simulink model "IDC_OS"  (R2023b)
settings: Solver=FixedStepAuto  StartTime=0.0  StopTime=9  FixedStep=sampleTime  RelTol=1e-3
values from neighbouring files (symbols this model uses):
  initialguess = robot.homeConfiguration    [IDC_OS.m]
  K_D = 0*eye(n_joints)    [IDC_OS.m]
  K_P = 0*eye(n_joints)    [IDC_OS.m]
  n_joints = 6    [IDC_OS.m]
  robot = loadrobot("universalUR5")    [IDC_OS.m]
  t0 = 0    [IDC_OS.m]
  t1 = 5    [IDC_OS.m]
  t2 = 10    [IDC_OS.m]
  t3 = 100    [IDC_OS.m]
  weights = transpose([0.1, 0.1, 0.1, 1, 1, 1])    [IDC_OS.m]
  x0_pose = trvec2tform([x0(1), x0(2), x0(3)]) * eul2tform([x0(4), x0(5), x0(6)])    [IDC_OS.m]
  xd = zeros(n_joints,1)    [IDC_OS.m]
undefined symbols (not defined in the file or in its folder): x1_pose, x2_pose
libraries: robotmaniplib x8
(part 2 of 2)

== matlab function IDC_OS/J_A^(-1)(q)*[...]/Analytical Jacobian/Analytical from Geometric ==
  data: geomJ input; Ja output; angles input
function Ja = JacobAnFromGeomWrapper(geomJ,angles)
% For T^-1 matrix using RPY i.e., z(r) y(p) x(y) wrt to the current frame

T = rpy2Tmatrix(angles);

Tinv = inv(T);

% Following matlab convention (Jo is on top of Jp)
Ja = [Tinv,zeros(3);zeros(3),eye(3)] * geomJ;

% In standard convention one would have:
% analytJ = [eye(3),zeros(3);zeros(3),Tinv] * geomJ;

== matlab function IDC_OS/J_A^(-1)(q)*[...]/Analytical Jacobian/Direct Kinematics/get RPY angles ==
  data: R input; rpy output
function rpy = rpyWrap(R)
%rpy = getRPYanglesFromR(R);
[rpy, ~] = eulerInverseProblem(R,'zyx','current');

== matlab function IDC_OS/J_A(q)*q./Analytical Jacobian/Direct Kinematics/get RPY angles ==
  data: R input; rpy output
function rpy = rpyWrap(R)
%rpy = getRPYanglesFromR(R);
[rpy, ~] = eulerInverseProblem(R,'zyx','current');

== matlab function IDC_OS/J_A^(-1)(q)*[...]/inverse ==
  data: u input; y output
function y = fcn(u)

y = pinv(u);

== matlab function IDC_OS/J_A(q)*q./Analytical Jacobian/Analytical from Geometric ==
  data: geomJ input; Ja output; angles input
function Ja = JacobAnFromGeomWrapper(geomJ,angles)
% For T^-1 matrix using RPY i.e., z(r) y(p) x(y) wrt to the current frame

T = rpy2Tmatrix(angles);

Tinv = inv(T);

% Following matlab convention (Jo is on top of Jp)
Ja = [Tinv,zeros(3);zeros(3),eye(3)] * geomJ;

% In standard convention one would have:
% analytJ = [eye(3),zeros(3);zeros(3),Tinv] * geomJ;

== matlab function IDC_OS/Forward Kinematics K(q)/Direct Kinematics/get RPY angles ==
  data: R input; rpy output
function rpy = rpyWrap(R)
%rpy = getRPYanglesFromR(R);
[rpy, ~] = eulerInverseProblem(R,'zyx','current');

== matlab function IDC_OS/Manipulator/J_A^(-1)(q)*[...]/Analytical Jacobian/Analytical from Geometric ==
  data: geomJ input; Ja output; angles input
function Ja = JacobAnFromGeomWrapper(geomJ,angles)
% For T^-1 matrix using RPY i.e., z(r) y(p) x(y) wrt to the current frame

T = rpy2Tmatrix(angles);

Tinv = inv(T);

% Following matlab convention (Jo is on top of Jp)
Ja = [Tinv,zeros(3);zeros(3),eye(3)] * geomJ;

% In standard convention one would have:
% analytJ = [eye(3),zeros(3);zeros(3),Tinv] * geomJ;

== matlab function IDC_OS/Manipulator/J_A^(-1)(q)*[...]/Analytical Jacobian/Direct Kinematics/get RPY angles ==
  data: R input; rpy output
function rpy = rpyWrap(R)
%rpy = getRPYanglesFromR(R);
[rpy, ~] = eulerInverseProblem(R,'zyx','current');

== matlab function IDC_OS/J._A(q,q.)*q./Analytical Jacobian/Analytical from Geometric ==
  data: geomJ input; Ja output; angles input
function Ja = JacobAnFromGeomWrapper(geomJ,angles)
% For T^-1 matrix using RPY i.e., z(r) y(p) x(y) wrt to the current frame

T = rpy2Tmatrix(angles);

Tinv = inv(T);

% Following matlab convention (Jo is on top of Jp)
Ja = [Tinv,zeros(3);zeros(3),eye(3)] * geomJ;

% In standard convention one would have:
% analytJ = [eye(3),zeros(3);zeros(3),Tinv] * geomJ;

== matlab function IDC_OS/J._A(q,q.)*q./Analytical Jacobian/Direct Kinematics/get RPY angles ==
  data: R input; rpy output
function rpy = rpyWrap(R)
%rpy = getRPYanglesFromR(R);
[rpy, ~] = eulerInverseProblem(R,'zyx','current');

== matlab function IDC_OS/Trajectory/5th poly PNP ==
  data: q_i input; q output; q_f input; t_i input; t_f input; t input
function q = fcn(q_i, q_f, t_i, t_f, t)

q = poly5PnP(q_i, q_f, t_i, t_f, t);
